simulink model "QuyDao"  (R2016a)
settings: Solver=ode45  StartTime=0.0  StopTime=322  RelTol=1e-3
values from neighbouring files (symbols this model uses):
  s = [s; t E]    [quydao.m]
libraries: mblibv1 x18
settings Model: Creator=Administrator  LastModifiedBy=Nam Nguyen
settings DataIOCC: LimitDataPoints=on  SaveFormat=Array
settings HardwareCC: ProdBitPerPointer=32  ProdLargestAtomicFloat=None  ProdIntDivRoundTo=Undefined  ProdEndianess=Unspecified  ProdWordSize=32  ProdHWDeviceType=32-bit Generic
settings ModelReferenceCC: PropagateSignalLabelsOutOfModel=off
settings ConfigComp: CovModelRefEnable=Off
settings SimMechanicsCC: VisOnUpdateDiagram=on  VisDuringSimulation=on
settings ConfigurationSet: Description=SimMechanics 2G

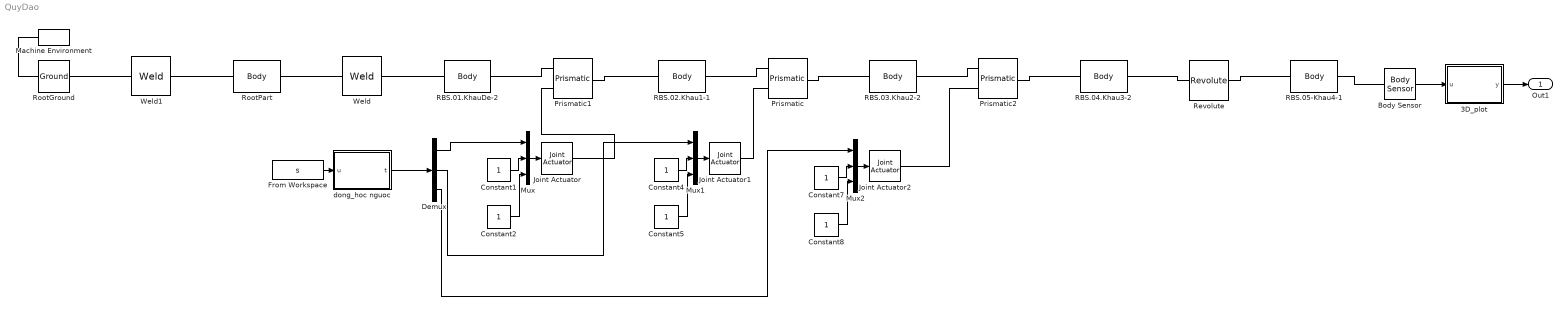
== system QuyDao ==
  3D_plot : MATLAB Function  TreatAsAtomicUnit=on
  Body Sensor : mblibv1/Sensors &  Actuators/Body Sensor  UpdateFromCAD=off  PhysicalDomain=Mechanical  PortType=blob  Muxed=on  Pose=off  Angle=on  AngleUnits=deg  ArcVelocity=off  ArcVelocityUnits=deg/s  ArcAcceleration=off  ArcAccelerationUnits=deg/s^2  CoordPosition=on  CoordPositionUnits=mm  Velocity=off  VelocityUnits=m/s  Acceleration=off  AccelerationUnits=m/s^2  Quaternion=on  QuaternionDT=off  QuaternionDDT=off  QuaternionUnits=off  OutputVector=[1]  ActiveIO=on  Width=3  DialogClass=MechanicalSensorBlock  ReferenceFrame=Absolute (World)
  Constant{1..2,4..5,7..8} (6 alike) : Constant
  Demux : Demux  Outputs=3
  From Workspace : FromWorkspace  VariableName=s  SampleTime=0.4
  Joint Actuator : mblibv1/Sensors &  Actuators/Joint Actuator  UpdateFromCAD=off  PhysicalDomain=Mechanical  PortType=blob  ActuationStyle=Motion  AngleUnits=deg  ArcVelocityUnits=deg/s  ArcAccelerationUnits=deg/s^2  CoordPositionUnits=mm  VelocityUnits=m/s  AccelerationUnits=m/s^2  ForceUnits=N  TorqueUnits=N*m  ActiveIO=on  Width=3  DialogClass=MechanicalActuatorBlock  Primitive=P1  ReferenceFrame=Absolute (World)
  Joint Actuator1 : mblibv1/Sensors &  Actuators/Joint Actuator  UpdateFromCAD=off  PhysicalDomain=Mechanical  PortType=blob  ActuationStyle=Motion  AngleUnits=deg  ArcVelocityUnits=deg/s  ArcAccelerationUnits=deg/s^2  CoordPositionUnits=mm  VelocityUnits=m/s  AccelerationUnits=m/s^2  ForceUnits=N  TorqueUnits=N*m  ActiveIO=on  Width=3  DialogClass=MechanicalActuatorBlock  Primitive=P1  ReferenceFrame=Absolute (World)
  Joint Actuator2 : mblibv1/Sensors &  Actuators/Joint Actuator  UpdateFromCAD=off  PhysicalDomain=Mechanical  PortType=blob  ActuationStyle=Motion  AngleUnits=deg  ArcVelocityUnits=deg/s  ArcAccelerationUnits=deg/s^2  CoordPositionUnits=mm  VelocityUnits=m/s  AccelerationUnits=m/s^2  ForceUnits=N  TorqueUnits=N*m  ActiveIO=on  Width=3  DialogClass=MechanicalActuatorBlock  Primitive=P1  ReferenceFrame=Absolute (World)
  Machine Environment : mblibv1/Bodies/Machine Environment  PortType=env  PhysicalDomain=Mechanical  DialogTemplateClass=MECH.MachineEnvironment  SyncWhenCopied=off  Gravity=[0 -9.81 0]  GravityUnits=m/s^2  GravityAsSignal=off  Dimensionality=Auto-detect  AnalysisType=Forward dynamics  LinearAssemblyTolerance=1e-3  LinearAssemblyToleranceUnits=m  AngularAssemblyTolerance=1e-3  AngularAssemblyToleranceUnits=rad  ConstraintSolverType=Stabilizing  ConstraintRelTolerance=1e-4  ConstraintAbsTolerance=1e-4  UseRobustSingularityHandling=off  RedundancyAnalysisToleranceType=Automatically select tolerance  RedundancyAnalysisTolerance=1e-14  StatePerturbationType=Fixed  PerturbationSize=1e-5  VisualizeMachine=on  BodyVisualizationType=Use model default body geometries  BodyColorSelMode=Use model default  DefaultBodyColor=[1 0 0]
  Mux : Mux  Inputs=3
  Mux1 : Mux  Inputs=3
  Mux2 : Mux  Inputs=3
  Prismatic : mblibv1/Joints/Prismatic  LConnTagsString=__newl0|SA1  RConnTagsString=__newr0  UpdateFromCAD=on  NumSAPorts=1  CutJoint=off  MarkAsCut=off  Primitives=prismatic  PrimitiveProps=P1$World$[-1,0,0]$prismatic  DialogClass=JointBlock  P1Axis=[-1,0,0]
  Prismatic1 : mblibv1/Joints/Prismatic  LConnTagsString=__newl0|SA1  RConnTagsString=__newr0  UpdateFromCAD=on  NumSAPorts=1  CutJoint=off  MarkAsCut=off  Primitives=prismatic  PrimitiveProps=P1$World$[0,0,1]$prismatic  DialogClass=JointBlock  P1Axis=[0,0,1]
  Prismatic2 : mblibv1/Joints/Prismatic  LConnTagsString=__newl0|SA1  RConnTagsString=__newr0  UpdateFromCAD=on  NumSAPorts=1  CutJoint=off  MarkAsCut=off  Primitives=prismatic  PrimitiveProps=P1$World$[0,-1,0]$prismatic  DialogClass=JointBlock  P1Axis=[0,-1,0]
  RBS.01.KhauDe-2 : mblibv1/Bodies/Body  LConnTagsString=CS2  RConnTagsString=CS3  UpdateFromCAD=on  DialogClass=MechanicalBodyBlock  Mass=0.481266  MassUnits=kg  InertiaUnits=kg*m^2  Inertia=[3.26313,0,0;0,3.76071,0;0,0,1.18222]  Shape=Cylinder  ShapeDims=[1 1]  ShapeUnits=m  ShapeUse=false  Density=1  DensityUnits=kg/m^3  DensityUse=false  GraphicsMode=GFXFILE  GraphicsFileName=sualai - RBS.01.KhauDe-2.STL  BodyColorSelMode=COLORPALETTE  BodyColor=[0.65098;0.619608;0.588235]  AttachedToCS=CS1  CG=Right$CG$[1.35 0.730871 2.35]$WORLD$WORLD$m$[1 0 0;0 1 0;0 0 1]$3x3 Transform$rad$WORLD$false$none  WorkingFrames=Right$CS1$[0 0 0]$WORLD$WORLD$m$[1 0 0;0 1 0;0 0 1]$3x3 Transform$rad$WORLD$false$none#Left$CS2$[1.35 0.730871 2.35]$WORLD$WORLD$m$[1 0 0;0 1 0;0 0 1]$3x3 Transform$rad$WORLD$true$none#Right$CS3$[0.283311 0.05 2.89491]$WORLD$WORLD$m$[1 0 0;0 1 0;0 0 1]$3x3 Transform$rad$WORLD$true$none  CGPos=[1.35 0.730871 2.35]  CGRot=[1 0 0;0 1 0;0 0 1]  CS0Pos=[]  CS0Rot=[]  CS1Pos=[0 0 0]  CS1Rot=[1 0 0;0 1 0;0 0 1]  CS2Pos=[1.35 0.730871 2.35]  CS2Rot=[1 0 0;0 1 0;0 0 1]  CS3Pos=[0.283311 0.05 2.89491]  CS3Rot=[1 0 0;0 1 0;0 0 1]  CS4Pos=[]  CS4Rot=[]  CS5Pos=[]  CS5Rot=[]  CS6Pos=[]  CS6Rot=[]  CS7Pos=[]  CS7Rot=[]  CS8Pos=[]  CS8Rot=[]  CS9Pos=[]  CS9Rot=[]  CS10Pos=[]  CS10Rot=[]  CS11Pos=[]  CS11Rot=[]  CS12Pos=[]  CS12Rot=[]  CS13Pos=[]  CS13Rot=[]  CS14Pos=[]  CS14Rot=[]  CS15Pos=[]  CS15Rot=[]  CS16Pos=[]  CS16Rot=[]  CS17Pos=[]  CS17Rot=[]  CS18Pos=[]  CS18Rot=[]  CS19Pos=[]  CS19Rot=[]  CS20Pos=[]  CS20Rot=[]
  RBS.02.Khau1-1 : mblibv1/Bodies/Body  LConnTagsString=CS3  RConnTagsString=CS2  UpdateFromCAD=on  DialogClass=MechanicalBodyBlock  Mass=0.091  MassUnits=kg  InertiaUnits=kg*m^2  Inertia=[0.0767067,0,0;0,0.0683701,0;0,0,0.00850512]  Shape=Cylinder  ShapeDims=[1 1]  ShapeUnits=m  ShapeUse=false  Density=1  DensityUnits=kg/m^3  DensityUse=false  GraphicsMode=GFXFILE  GraphicsFileName=sualai - RBS.02.Khau1-1.STL  BodyColorSelMode=COLORPALETTE  BodyColor=[0.65098;0.619608;0.588235]  AttachedToCS=CS1  CG=Right$CG$[1.35 -0.0387363 1.523]$WORLD$WORLD$m$[0 0 1;-1 0 0;0 -1 0]$3x3 Transform$rad$WORLD$false$none  WorkingFrames=Right$CS1$[0.2 -0.1 1.523]$WORLD$WORLD$m$[0 0 1;-1 0 0;0 -1 0]$3x3 Transform$rad$WORLD$false$none#Right$CS2$[0.44375 -0.1 1.35269]$WORLD$WORLD$m$[1 0 0;0 1 0;0 0 1]$3x3 Transform$rad$WORLD$true$none#Left$CS3$[0.283311 0.05 2.89491]$WORLD$WORLD$m$[1 0 0;0 1 0;0 0 1]$3x3 Transform$rad$WORLD$true$none  CGPos=[1.35 -0.0387363 1.523]  CGRot=[0 0 1;-1 0 0;0 -1 0]  CS0Pos=[]  CS0Rot=[]  CS1Pos=[0.2 -0.1 1.523]  CS1Rot=[0 0 1;-1 0 0;0 -1 0]  CS2Pos=[0.44375 -0.1 1.35269]  CS2Rot=[1 0 0;0 1 0;0 0 1]  CS3Pos=[0.283311 0.05 2.89491]  CS3Rot=[1 0 0;0 1 0;0 0 1]  CS4Pos=[]  CS4Rot=[]  CS5Pos=[]  CS5Rot=[]  CS6Pos=[]  CS6Rot=[]  CS7Pos=[]  CS7Rot=[]  CS8Pos=[]  CS8Rot=[]  CS9Pos=[]  CS9Rot=[]  CS10Pos=[]  CS10Rot=[]  CS11Pos=[]  CS11Rot=[]  CS12Pos=[]  CS12Rot=[]  CS13Pos=[]  CS13Rot=[]  CS14Pos=[]  CS14Rot=[]  CS15Pos=[]  CS15Rot=[]  CS16Pos=[]  CS16Rot=[]  CS17Pos=[]  CS17Rot=[]  CS18Pos=[]  CS18Rot=[]  CS19Pos=[]  CS19Rot=[]  CS20Pos=[]  CS20Rot=[]
  RBS.03.Khau2-2 : mblibv1/Bodies/Body  LConnTagsString=CS2  RConnTagsString=CS3  UpdateFromCAD=on  DialogClass=MechanicalBodyBlock  Mass=678.24  MassUnits=kg  InertiaUnits=kg*m^2  Inertia=[193.644,0,0;0,196.51,-6.39404;0,-6.39404,12.4099]  Shape=Cylinder  ShapeDims=[1 1]  ShapeUnits=m  ShapeUse=false  Density=1  DensityUnits=kg/m^3  DensityUse=false  GraphicsMode=GFXFILE  GraphicsFileName=sualai - RBS.03.Khau2-2.STL  BodyColorSelMode=COLORPALETTE  BodyColor=[1 0 0]  AttachedToCS=CS1  CG=Right$CG$[0.623217 -0.135278 1.523]$WORLD$WORLD$m$[0 1 0;0 0 1;1 0 0]$3x3 Transform$rad$WORLD$false$none  WorkingFrames=Right$CS1$[0.809559 -1.09 1.523]$WORLD$WORLD$m$[0 1 0;0 0 1;1 0 0]$3x3 Transform$rad$WORLD$false$none#Left$CS2$[0.44375 -0.1 1.35269]$WORLD$WORLD$m$[1 0 0;0 1 0;0 0 1]$3x3 Transform$rad$WORLD$true$none#Right$CS3$[0.709559 -0.75 1.423]$WORLD$WORLD$m$[1 0 0;0 1 0;0 0 1]$3x3 Transform$rad$WORLD$true$none  CGPos=[0.623217 -0.135278 1.523]  CGRot=[0 1 0;0 0 1;1 0 0]  CS0Pos=[]  CS0Rot=[]  CS1Pos=[0.809559 -1.09 1.523]  CS1Rot=[0 1 0;0 0 1;1 0 0]  CS2Pos=[0.44375 -0.1 1.35269]  CS2Rot=[1 0 0;0 1 0;0 0 1]  CS3Pos=[0.709559 -0.75 1.423]  CS3Rot=[1 0 0;0 1 0;0 0 1]  CS4Pos=[]  CS4Rot=[]  CS5Pos=[]  CS5Rot=[]  CS6Pos=[]  CS6Rot=[]  CS7Pos=[]  CS7Rot=[]  CS8Pos=[]  CS8Rot=[]  CS9Pos=[]  CS9Rot=[]  CS10Pos=[]  CS10Rot=[]  CS11Pos=[]  CS11Rot=[]  CS12Pos=[]  CS12Rot=[]  CS13Pos=[]  CS13Rot=[]  CS14Pos=[]  CS14Rot=[]  CS15Pos=[]  CS15Rot=[]  CS16Pos=[]  CS16Rot=[]  CS17Pos=[]  CS17Rot=[]  CS18Pos=[]  CS18Rot=[]  CS19Pos=[]  CS19Rot=[]  CS20Pos=[]  CS20Rot=[]
  RBS.04.Khau3-2 : mblibv1/Bodies/Body  LConnTagsString=CS2  RConnTagsString=CS3  UpdateFromCAD=on  DialogClass=MechanicalBodyBlock  Mass=363.732  MassUnits=kg  InertiaUnits=kg*m^2  Inertia=[108.563,0,0;0,108.563,0;0,0,3.30044]  Shape=Cylinder  ShapeDims=[1 1]  ShapeUnits=m  ShapeUse=false  Density=1  DensityUnits=kg/m^3  DensityUse=false  GraphicsMode=GFXFILE  GraphicsFileName=sualai - RBS.04.Khau3-2.STL  BodyColorSelMode=COLORPALETTE  BodyColor=[0;1;1]  AttachedToCS=CS1  CG=Right$CG$[0.809559 1.1517 1.523]$WORLD$WORLD$m$[0 1 0;0 0 1;1 0 0]$3x3 Transform$rad$WORLD$false$none  WorkingFrames=Right$CS1$[0.809559 2.0111 1.523]$WORLD$WORLD$m$[0 1 0;0 0 1;1 0 0]$3x3 Transform$rad$WORLD$false$none#Left$CS2$[0.709559 -0.75 1.423]$WORLD$WORLD$m$[1 0 0;0 1 0;0 0 1]$3x3 Transform$rad$WORLD$true$none#Right$CS3$[0.809559 2.0111 1.523]$WORLD$WORLD$m$[1 0 0;0 1 0;0 0 1]$3x3 Transform$rad$WORLD$true$none  CGPos=[0.809559 1.1517 1.523]  CGRot=[0 1 0;0 0 1;1 0 0]  CS0Pos=[]  CS0Rot=[]  CS1Pos=[0.809559 2.0111 1.523]  CS1Rot=[0 1 0;0 0 1;1 0 0]  CS2Pos=[0.709559 -0.75 1.423]  CS2Rot=[1 0 0;0 1 0;0 0 1]  CS3Pos=[0.809559 2.0111 1.523]  CS3Rot=[1 0 0;0 1 0;0 0 1]  CS4Pos=[]  CS4Rot=[]  CS5Pos=[]  CS5Rot=[]  CS6Pos=[]  CS6Rot=[]  CS7Pos=[]  CS7Rot=[]  CS8Pos=[]  CS8Rot=[]  CS9Pos=[]  CS9Rot=[]  CS10Pos=[]  CS10Rot=[]  CS11Pos=[]  CS11Rot=[]  CS12Pos=[]  CS12Rot=[]  CS13Pos=[]  CS13Rot=[]  CS14Pos=[]  CS14Rot=[]  CS15Pos=[]  CS15Rot=[]  CS16Pos=[]  CS16Rot=[]  CS17Pos=[]  CS17Rot=[]  CS18Pos=[]  CS18Rot=[]  CS19Pos=[]  CS19Rot=[]  CS20Pos=[]  CS20Rot=[]
  RBS.05-Khau4-1 : mblibv1/Bodies/Body  LConnTagsString=CS2  RConnTagsString=CS1  UpdateFromCAD=on  DialogClass=MechanicalBodyBlock  Mass=26.144  MassUnits=kg  InertiaUnits=kg*m^2  Inertia=[0.122087,0,0;0,0.139242,0;0,0,0.219027]  Shape=Cylinder  ShapeDims=[1 1]  ShapeUnits=m  ShapeUse=false  Density=1  DensityUnits=kg/m^3  DensityUse=false  GraphicsMode=GFXFILE  GraphicsFileName=sualai - RBS.05-Khau4-1.STL  BodyColorSelMode=COLORPALETTE  BodyColor=[1 1 0]  AttachedToCS=CS1  CG=Right$CG$[0.809498 2.0611 1.52775]$WORLD$WORLD$m$[-0.0129085 0.999917 0;0 0 1;0.999917 0.0129085 0]$3x3 Transform$rad$WORLD$false$none  WorkingFrames=Right$CS1$[0.806332 2.0611 1.77298]$WORLD$WORLD$m$[-0.0129085 0.999917 0;0 0 1;0.999917 0.0129085 0]$3x3 Transform$rad$WORLD$true$none#Left$CS2$[0.809559 2.0111 1.523]$WORLD$WORLD$m$[1 0 0;0 1 0;0 0 1]$3x3 Transform$rad$WORLD$true$none  CGPos=[0.809498 2.0611 1.52775]  CGRot=[-0.0129085 0.999917 0;0 0 1;0.999917 0.0129085 0]  CS0Pos=[]  CS0Rot=[]  CS1Pos=[0.806332 2.0611 1.77298]  CS1Rot=[-0.0129085 0.999917 0;0 0 1;0.999917 0.0129085 0]  CS2Pos=[0.809559 2.0111 1.523]  CS2Rot=[1 0 0;0 1 0;0 0 1]  CS3Pos=[]  CS3Rot=[]  CS4Pos=[]  CS4Rot=[]  CS5Pos=[]  CS5Rot=[]  CS6Pos=[]  CS6Rot=[]  CS7Pos=[]  CS7Rot=[]  CS8Pos=[]  CS8Rot=[]  CS9Pos=[]  CS9Rot=[]  CS10Pos=[]  CS10Rot=[]  CS11Pos=[]  CS11Rot=[]  CS12Pos=[]  CS12Rot=[]  CS13Pos=[]  CS13Rot=[]  CS14Pos=[]  CS14Rot=[]  CS15Pos=[]  CS15Rot=[]  CS16Pos=[]  CS16Rot=[]  CS17Pos=[]  CS17Rot=[]  CS18Pos=[]  CS18Rot=[]  CS19Pos=[]  CS19Rot=[]  CS20Pos=[]  CS20Rot=[]
  Revolute : mblibv1/Joints/Revolute  LConnTagsString=__newl0  RConnTagsString=__newr0  UpdateFromCAD=on  NumSAPorts=0  CutJoint=off  MarkAsCut=off  Primitives=prismatic  PrimitiveProps=R1$World$[0,1,0]$revolute  DialogClass=JointBlock  R1Axis=[0,1,0]
  RootGround : mblibv1/Bodies/Ground  UpdateFromCAD=on  LeftPortType=env  RightPortType=workingframe  PhysicalDomain=Mechanical  DialogClass=GroundBlock  CoordPosition=[1.22346,0.560132,2.08492]  CoordPositionUnits=m  StateVectorMgrId=-1  MachineId=[0 0]  ShowEnvPort=on  ParameterChecksum=[3472440782, 3200816749, 389633693, 530832971]  TopologyChecksum=[833561479, 3092682974, 2234461456, 99938200]
  RootPart : mblibv1/Bodies/Body  LConnTagsString=CS3  RConnTagsString=CS2  UpdateFromCAD=on  DialogClass=MechanicalBodyBlock  Mass=0  MassUnits=kg  InertiaUnits=kg*m^2  Inertia=[0,0,0;0,0,0;0,0,0]  Shape=Cylinder  ShapeDims=[1 1]  ShapeUnits=m  ShapeUse=false  Density=1  DensityUnits=kg/m^3  DensityUse=false  GraphicsMode=MACHINE_DEFAULT  BodyColorSelMode=MACHINE_DEFAULT  BodyColor=[1;0;0]  AttachedToCS=CS1  CG=Right$CG$[1.22346 0.560132 2.08492]$WORLD$WORLD$m$[1 0 0;0 1 0;0 0 1]$3x3 Transform$rad$WORLD$false$none  WorkingFrames=Right$CS1$[0 0 0]$WORLD$WORLD$m$[1 0 0;0 1 0;0 0 1]$3x3 Transform$rad$WORLD$false$none#Right$CS2$[1.35 0.730871 2.35]$WORLD$WORLD$m$[1 0 0;0 1 0;0 0 1]$3x3 Transform$rad$WORLD$true$none#Left$CS3$[1.22346 0.560132 2.08492]$WORLD$WORLD$m$[1 0 0;0 1 0;0 0 1]$3x3 Transform$rad$WORLD$true$none  CGPos=[1.22346 0.560132 2.08492]  CGRot=[1 0 0;0 1 0;0 0 1]  CS0Pos=[]  CS0Rot=[]  CS1Pos=[0 0 0]  CS1Rot=[1 0 0;0 1 0;0 0 1]  CS2Pos=[1.35 0.730871 2.35]  CS2Rot=[1 0 0;0 1 0;0 0 1]  CS3Pos=[1.22346 0.560132 2.08492]  CS3Rot=[1 0 0;0 1 0;0 0 1]  CS4Pos=[]  CS4Rot=[]  CS5Pos=[]  CS5Rot=[]  CS6Pos=[]  CS6Rot=[]  CS7Pos=[]  CS7Rot=[]  CS8Pos=[]  CS8Rot=[]  CS9Pos=[]  CS9Rot=[]  CS10Pos=[]  CS10Rot=[]  CS11Pos=[]  CS11Rot=[]  CS12Pos=[]  CS12Rot=[]  CS13Pos=[]  CS13Rot=[]  CS14Pos=[]  CS14Rot=[]  CS15Pos=[]  CS15Rot=[]  CS16Pos=[]  CS16Rot=[]  CS17Pos=[]  CS17Rot=[]  CS18Pos=[]  CS18Rot=[]  CS19Pos=[]  CS19Rot=[]  CS20Pos=[]  CS20Rot=[]
  Weld : mblibv1/Joints/Weld  LConnTagsString=__newl0  RConnTagsString=__newr0  UpdateFromCAD=on  NumSAPorts=0  CutJoint=off  MarkAsCut=off  Primitives=weld  PrimitiveProps=W$WORLD$[0.57735,0.57735,0.57735]$weld  DialogClass=JointBlock  WAxis=[0.57735,0.57735,0.57735]
  Weld1 : mblibv1/Joints/Weld  LConnTagsString=__newl0  RConnTagsString=__newr0  UpdateFromCAD=on  NumSAPorts=0  CutJoint=off  MarkAsCut=off  Primitives=weld  PrimitiveProps=W$WORLD$[0.57735,0.57735,0.57735]$weld  DialogClass=JointBlock  WAxis=[0.57735,0.57735,0.57735]
  dong_hoc nguoc : MATLAB Function  TreatAsAtomicUnit=on
  Out1 : Outport
  wires:
  Demux/1 -> Mux/1
  Constant1/1 -> Mux/2
  Constant2/1 -> Mux/3
  Mux/1 -> Joint Actuator/1
  Demux/2 -> Mux1/1
  Constant4/1 -> Mux1/2
  Constant5/1 -> Mux1/3
  Mux1/1 -> Joint Actuator1/1
  Demux/3 -> Mux2/1
  Constant7/1 -> Mux2/2
  Constant8/1 -> Mux2/3
  Mux2/1 -> Joint Actuator2/1
  dong_hoc nguoc/1(t) -> Demux/1
  Body Sensor/1 -> 3D_plot/1(u)
  3D_plot/1(y) -> Out1/1
  From Workspace/1 -> dong_hoc nguoc/1(u)
  connections:
  Body Sensor/LConn1 -- RBS.05-Khau4-1/RConn1
  RootPart/RConn1 -- Weld/LConn1
  RootGround/LConn1 -- Machine Environment/RConn1
  Weld/RConn1 -- RBS.01.KhauDe-2/LConn1
  Revolute/RConn1 -- RBS.05-Khau4-1/LConn1
  Prismatic/RConn1 -- RBS.03.Khau2-2/LConn1
  RootGround/RConn1 -- Weld1/LConn1
  RBS.03.Khau2-2/RConn1 -- Prismatic2/LConn1
  Prismatic2/RConn1 -- RBS.04.Khau3-2/LConn1
  RBS.01.KhauDe-2/RConn1 -- Prismatic1/LConn1
  Prismatic1/RConn1 -- RBS.02.Khau1-1/LConn1
  Weld1/RConn1 -- RootPart/LConn1
  RBS.04.Khau3-2/RConn1 -- Revolute/LConn1
  RBS.02.Khau1-1/RConn1 -- Prismatic/LConn1
  Joint Actuator/RConn1 -- Prismatic1/LConn2
  Joint Actuator1/RConn1 -- Prismatic/LConn2
  Joint Actuator2/RConn1 -- Prismatic2/LConn2

== matlab function QuyDao/3D_plot ==
  data: u input; y output
function y = fcn(u)
%#codegen
x1=u(1,1)
x2=u(2,1)
x3=u(3,1)
plot3(-x3,x2,x1,'b.');
hold on;
grid on
y = u;

== matlab function QuyDao/dong_hoc nguoc ==
  data: u input; t output
function t = fcn(u)
%#codegen
x=u(1);
y=u(2);
z=u(3);
vx=u(4);
vy=u(5);
vz=u(6);
ax=u(7);
ay=u(8);
az=u(9)
d1=60;
d2=360;
d3=620;
a3=110;
t1=z-d1;
t2=-x+d2-a3;
t3=-y-d3;

t1_dot=vz;
t2_dot=-vx;
t3_dot=-vy;

t1_2dot=az;
t2_2dot=-ax;
t3_2dot=-ay;
t=[t1 t2 t3 ]
